simulink model "untitled"  (Simulink 8.0)
settings: Solver=ode45  StartTime=0.0  StopTime=10  RelTol=1e-3
values from neighbouring files (symbols this model uses):
  den_k = [1 100*a]    [Sve_ikad.m]
  Kp = 41.55    [Sve_ikad.m]    (also in matlab.mat = 41.6)
  num_k = [1*a 100]    [Sve_ikad.m]
settings Model: Creator=Labos  LastModifiedBy=Niko
settings DataIOCC: SignalLoggingSaveFormat=ModelDataLogs
settings DebuggingCC: FcnCallInpInsideContextMsg=UseLocalSettings  StrictBusMsg=Warning
settings GRTTargetCC: CombineOutputUpdateFcns=off  GRTInterface=on

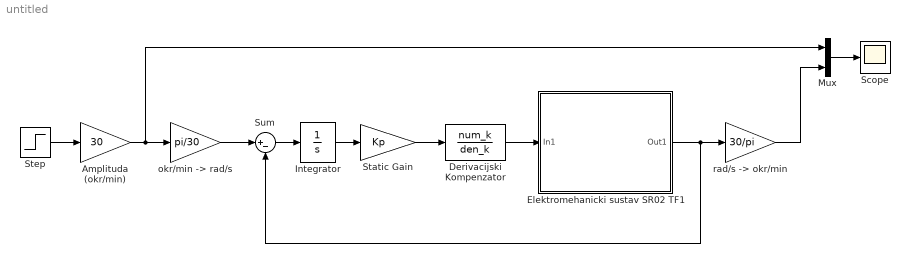
== system untitled ==
  Amplituda (okr/min) : Gain  Gain=30
  Derivacijski Kompenzator : TransferFcn  Numerator=num_k  Denominator=den_k
  Elektromehanicki sustav SR02 TF1 : Subsystem  mask{Ra=2.6, ke=0.0076776, km=0.007683, Jeq=9.785e-5, Beq=0.0015, Kg=14, ng=0.9, nm=0.69, w0=0}
      mask prompts: Ra "Otpor armature (Ra)"; ke "Konstanta protuelektromotorne sile (Ke)"; km "Konstanta momenta motora (Km)"; Jeq "Ekvivalentni moment tromosti kod opterecenja (Jeq)"; Beq "Ekvivalentni koeficjent viskoznog trenja Beq"; Kg "SRV02 omjer zupcanika sustava (Kg)"; ng "Korisnost zupcastog prijenosa (Eff_G)"; nm "Korisnost motora (EfF_M)"; w0 "Pocetna kutna brzina(w0)"
      mask help: Nadomjesni model elektromehanickog sustava SR02
      mask init:
      | Ra = 2.6
      | ke = 0.0076776
      | km = 0.007683
      | Jm = 33.87e-7
      | Jeq = 9.785e-5
      | Beq = 0.0015
      | Kg = 14
      | ng = 0.9
      | nm = 0.69
      mask Display:
      | port_label('input',1,'Ua')
      | port_label('output',1,'w')
  Integrator : Integrator
  Mux : Mux  Inputs=2
  Scope : Scope
      settings: SaveName=Response
  Static Gain : Gain  Gain=Kp
  Step : Step  SampleTime=0
  Sum : Sum  Inputs=|+-
  "okr/min -> rad/s" : Gain  Gain=pi/30
  "rad/s -> okr/min" : Gain  Gain=30/pi
  wires:
  Step/1 -> Amplituda (okr/min)/1
  Amplituda (okr/min)/1 -> Mux/1, "okr/min -> rad/s"/1
  "okr/min -> rad/s"/1 -> Sum/1
  Sum/1 -> Integrator/1
  Integrator/1 -> Static Gain/1
  Static Gain/1 -> Derivacijski Kompenzator/1
  Derivacijski Kompenzator/1 -> Elektromehanicki sustav SR02 TF1/1(In1)
  Elektromehanicki sustav SR02 TF1/1(Out1) -> Sum/2, "rad/s -> okr/min"/1
  "rad/s -> okr/min"/1 -> Mux/2
  Mux/1 -> Scope/1

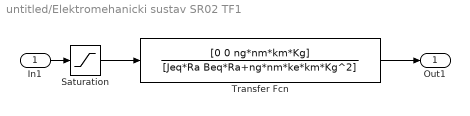
== system untitled/Elektromehanicki sustav SR02 TF1 ==
  In1 : Inport
  Saturation : Saturate  UpperLimit=6  LowerLimit=-6
  Transfer Fcn : TransferFcn  Numerator=[0 0 ng*nm*km*Kg]  Denominator=[Jeq*Ra Beq*Ra+ng*nm*ke*km*Kg^2]
  Out1 : Outport
  wires:
  Saturation/1 -> Transfer Fcn/1
  Transfer Fcn/1 -> Out1/1
  In1/1 -> Saturation/1
